simulink model "aae301hw08pg192"  (R2016a)
settings: Solver=VariableStepAuto  StartTime=0.0  StopTime=10.0  RelTol=1e-3
settings Model: Creator=mayer15  LastModifiedBy=mayer15

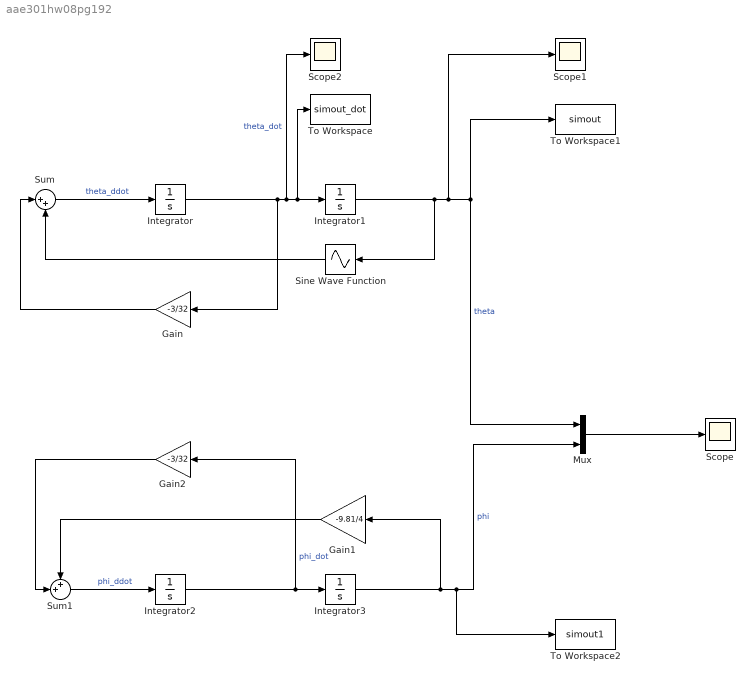
== system aae301hw08pg192 ==
  Gain : Gain  Gain=-3/32
  Gain1 : Gain  Gain=-9.81/4
  Gain2 : Gain  Gain=-3/32
  Integrator{,1..3} (4 alike) : Integrator
  Mux : Mux  Inputs=2
  Scope : Scope
  Scope1 : Scope
  Scope2 : Scope
  Sine Wave Function : Sin  TimeSource=Use external signal  Amplitude=-9.81/4  SampleTime=0
  Sum : Sum  Inputs=|++
  Sum1 : Sum  Inputs=++|
  To Workspace : ToWorkspace  VariableName=simout_dot  SaveFormat=Timeseries  SampleTime=-1
  To Workspace1 : ToWorkspace  VariableName=simout  SaveFormat=Timeseries  SampleTime=-1
  To Workspace2 : ToWorkspace  VariableName=simout1  SaveFormat=Timeseries  SampleTime=-1
  wires:
  Mux/1 -> Scope/1
  Integrator1/1 -> Sine Wave Function/1, Scope1/1, Mux/1, To Workspace1/1  "theta"
  Integrator/1 -> Gain/1, Scope2/1, To Workspace/1, Integrator1/1  "theta_dot"
  Sine Wave Function/1 -> Sum/2
  Gain/1 -> Sum/1
  Sum/1 -> Integrator/1  "theta_ddot"
  Integrator3/1 -> Gain1/1, To Workspace2/1, Mux/2  "phi"
  Integrator2/1 -> Gain2/1, Integrator3/1  "phi_dot"
  Gain1/1 -> Sum1/1
  Gain2/1 -> Sum1/2
  Sum1/1 -> Integrator2/1  "phi_ddot"
